simulink model "company"  (R2016b)
settings: Solver=ode4  StartTime=0.0  StopTime=100  FixedStep=0.01  RelTol=1e-3
settings Model: Creator=Thomas  LastModifiedBy=Thomas

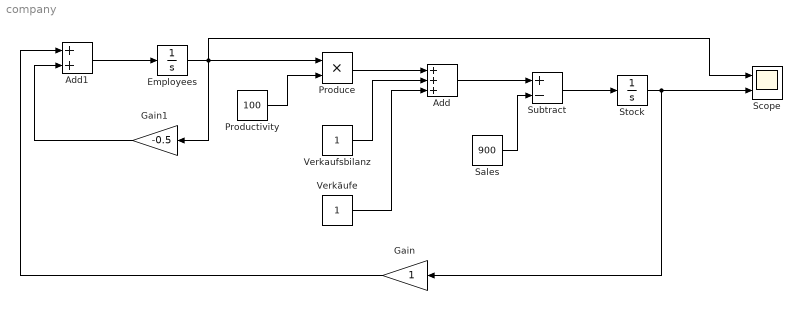
== system company ==
  Add : Sum  Inputs=+++
  Add1 : Sum
  Employees : Integrator  InitialCondition=1
  Gain : Gain
  Gain1 : Gain  Gain=-0.5
  Produce : Product
  Productivity : Constant  Value=100
  Sales : Constant  Value=900
  Scope : Scope  NumInputPorts=2
  Stock : Integrator
  Subtract : Sum  Inputs=+-
  Verkaufsbilanz : Constant
  Verkäufe : Constant
  wires:
  Productivity/1 -> Produce/2
  Employees/1 -> Scope/1, Gain1/1, Produce/1
  Produce/1 -> Add/1
  Verkaufsbilanz/1 -> Add/2
  Verkäufe/1 -> Add/3
  Stock/1 -> Scope/2, Gain/1
  Add1/1 -> Employees/1
  Gain1/1 -> Add1/2
  Add/1 -> Subtract/1
  Sales/1 -> Subtract/2
  Subtract/1 -> Stock/1
  Gain/1 -> Add1/1
